simulink model "SysGenBCM1CoreV2"  (R2015b)
settings: Solver=ode45  StartTime=0.0  StopTime=2e-3  MaxStep=100e-6  RelTol=1e-3
undefined symbols (not defined in the file): AXI4, Lite
libraries: xbsIndex_r4 x94
settings Model: DataTypeOverride=Double  MinMaxOverflowLogging=MinMaxAndOverflow  FPTRunName=DoubleOverride  Creator=ssmith  LastModifiedBy=leosap
settings DataIOCC: SaveFormat=Array
settings DebuggingCC: UnderspecifiedInitializationDetection=Classic  MergeDetectMultiDrivingBlocksExec=none  SolverPrmCheckMsg=warning
settings HardwareCC: ProdBitPerPointer=32  ProdLargestAtomicFloat=None  ProdIntDivRoundTo=Undefined  ProdEndianess=Unspecified  ProdWordSize=32  ProdHWDeviceType=32-bit Generic
settings GRTTargetCC: GeneratePreprocessorConditionals=Disable all
settings ConfigComp: CovModelRefEnable=Off  CovSFcnEnable=off

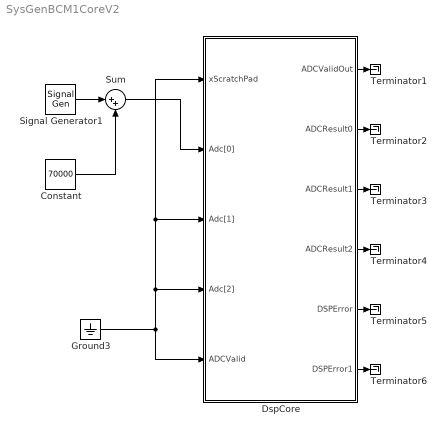
== system SysGenBCM1CoreV2 ==
  Constant : Constant  Value=70000
  DspCore : Subsystem
  Ground3 : Ground
  Signal Generator1 : SignalGenerator  Amplitude=65000  Frequency=1E+6  Units=rad/sec
  Sum : Sum  Inputs=|++
  Terminator{1..6} (6 alike) : Terminator
  wires:
  Ground3/1 -> DspCore/5(ADCValid), DspCore/3(Adc[1]), DspCore/1(xScratchPad), DspCore/4(Adc[2])
  Constant/1 -> Sum/2
  Signal Generator1/1 -> Sum/1
  DspCore/1(ADCValidOut) -> Terminator1/1
  DspCore/2(ADCResult0) -> Terminator2/1
  DspCore/3(ADCResult1) -> Terminator3/1
  DspCore/4(ADCResult2) -> Terminator4/1
  DspCore/5(DSPError) -> Terminator5/1
  DspCore/6(DSPError1) -> Terminator6/1
  Sum/1 -> DspCore/2(Adc[0])

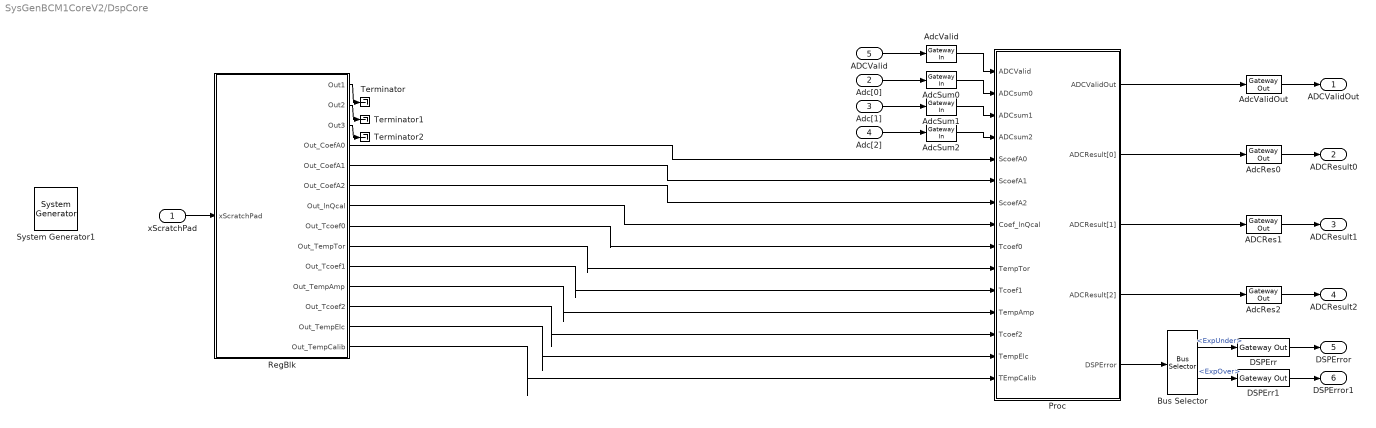
== system SysGenBCM1CoreV2/DspCore ==
  xScratchPad : Inport
  Adc[0] : Inport  Port=2
  Adc[1] : Inport  Port=3
  Adc[2] : Inport  Port=4
  ADCValid : Inport  Port=5
  " System Generator1" : xbsIndex_r4/ System Generator  Tag=genX  xilinxfamily=kintexu  part=xcku040  speed=-2-e  package=ffva1156  synthesis_tool=Vivado  clock_wrapper=Clock Enables  directory=./netlist  proj_type=Vivado  Synth_file=Vivado Synthesis Defaults  Impl_file=Vivado Implementation Defaults  testbench=off  simulink_period=5.385e-9  sysclk_period=5.385  dcm_input_clock_period=10  incr_netlist=off  trim_vbits=Everywhere in SubSystem  dbl_ovrd=According to Block Masks  core_generation=According to Block Masks  run_coregen=off  deprecated_control=off  eval_field=0  block_type=sysgen
  ADCRes1 : xbsIndex_r4/Gateway Out  inherit_from_input=on  hdl_port=on  rows=1  columns=1  UseAsDAC=off  DACChannel='1'  interface=None  automatic_assignment=on  address_offset=hex2dec('00')  intf_name=''  intf_description=''  timing_constraint=None  locs_specified=off  LOCs={}  io_standard={}  block_type=gatewayout
  AdcRes0 : xbsIndex_r4/Gateway Out  inherit_from_input=on  hdl_port=on  rows=1  columns=1  UseAsDAC=off  DACChannel='1'  interface=None  automatic_assignment=on  address_offset=hex2dec('00')  intf_name=''  intf_description=''  timing_constraint=None  locs_specified=off  LOCs={}  io_standard={}  block_type=gatewayout
  AdcRes2 : xbsIndex_r4/Gateway Out  inherit_from_input=on  hdl_port=on  rows=1  columns=1  UseAsDAC=off  DACChannel='1'  interface=None  automatic_assignment=on  address_offset=hex2dec('00')  intf_name=''  intf_description=''  timing_constraint=None  locs_specified=off  LOCs={}  io_standard={}  block_type=gatewayout
  AdcSum0 : xbsIndex_r4/Gateway In  gui_display_data_type=Fixed-point  arith_type=Unsigned  n_bits=32  bin_pt=0  preci_type=Single  exp_width=8  frac_width=24  rows=1  columns=1  quantization="Round  (unbiased: +/- Inf)"  overflow=Saturate  period=5.385E-9  UseAsADC=off  ADCChannel='1'  interface=None  automatic_assignment=on  address_offset=hex2dec('00')  intf_name=''  intf_description=''  default_value=0  timing_constraint=None  locs_specified=off  LOCs={}  io_standard={}  inherit_from_input=off  hdl_port=on  dbl_ovrd=off  block_type=gatewayin
  AdcSum1 : xbsIndex_r4/Gateway In  gui_display_data_type=Fixed-point  arith_type=Unsigned  n_bits=32  bin_pt=0  preci_type=Single  exp_width=8  frac_width=24  rows=1  columns=1  quantization="Round  (unbiased: +/- Inf)"  overflow=Saturate  period=5.385E-9  UseAsADC=off  ADCChannel='1'  interface=None  automatic_assignment=on  address_offset=hex2dec('00')  intf_name=''  intf_description=''  default_value=0  timing_constraint=None  locs_specified=off  LOCs={}  io_standard={}  inherit_from_input=off  hdl_port=on  dbl_ovrd=off  block_type=gatewayin
  AdcSum2 : xbsIndex_r4/Gateway In  gui_display_data_type=Fixed-point  arith_type=Unsigned  n_bits=32  bin_pt=0  preci_type=Single  exp_width=8  frac_width=24  rows=1  columns=1  quantization="Round  (unbiased: +/- Inf)"  overflow=Saturate  period=5.385E-9  UseAsADC=off  ADCChannel='1'  interface=None  automatic_assignment=on  address_offset=hex2dec('00')  intf_name=''  intf_description=''  default_value=0  timing_constraint=None  locs_specified=off  LOCs={}  io_standard={}  inherit_from_input=off  hdl_port=on  dbl_ovrd=off  block_type=gatewayin
  AdcValid : xbsIndex_r4/Gateway In  gui_display_data_type=Boolean  arith_type=Boolean  n_bits=1  bin_pt=0  preci_type=Single  exp_width=8  frac_width=24  rows=1  columns=1  quantization="Round  (unbiased: +/- Inf)"  overflow=Saturate  period=5.385E-9  UseAsADC=off  ADCChannel='1'  interface=None  automatic_assignment=on  address_offset=hex2dec('00')  intf_name=''  intf_description=''  default_value=0  timing_constraint=None  locs_specified=off  LOCs={}  io_standard={}  inherit_from_input=off  hdl_port=on  dbl_ovrd=off  block_type=gatewayin
  AdcValidOut : xbsIndex_r4/Gateway Out  inherit_from_input=on  hdl_port=on  rows=1  columns=1  UseAsDAC=off  DACChannel='1'  interface=None  automatic_assignment=on  address_offset=hex2dec('00')  intf_name=''  intf_description=''  timing_constraint=None  locs_specified=off  LOCs={}  io_standard={}  block_type=gatewayout
  Bus Selector : BusSelector  OutputSignals=ExpUnder,ExpOver
  DSPErr : xbsIndex_r4/Gateway Out  inherit_from_input=on  hdl_port=on  rows=1  columns=1  UseAsDAC=off  DACChannel='1'  interface=None  automatic_assignment=on  address_offset=hex2dec('00')  intf_name=''  intf_description=''  timing_constraint=None  locs_specified=off  LOCs={}  io_standard={}  block_type=gatewayout
  DSPErr1 : xbsIndex_r4/Gateway Out  inherit_from_input=on  hdl_port=on  rows=1  columns=1  UseAsDAC=off  DACChannel='1'  interface=None  automatic_assignment=on  address_offset=hex2dec('00')  intf_name=''  intf_description=''  timing_constraint=None  locs_specified=off  LOCs={}  io_standard={}  block_type=gatewayout
  Proc : Subsystem
  RegBlk : Subsystem
  Terminator : Terminator
  Terminator1 : Terminator
  Terminator2 : Terminator
  ADCValidOut : Outport
  ADCResult0 : Outport  Port=2
  ADCResult1 : Outport  Port=3
  ADCResult2 : Outport  Port=4
  DSPError : Outport  Port=5
  DSPError1 : Outport  Port=6
  wires:
  xScratchPad/1 -> RegBlk/1(xScratchPad)
  Proc/1(ADCValidOut) -> AdcValidOut/1
  Adc[2]/1 -> AdcSum2/1
  Adc[1]/1 -> AdcSum1/1
  Adc[0]/1 -> AdcSum0/1
  Proc/3(ADCResult[1]) -> ADCRes1/1
  Proc/4(ADCResult[2]) -> AdcRes2/1
  Proc/2(ADCResult[0]) -> AdcRes0/1
  ADCValid/1 -> AdcValid/1
  AdcRes0/1 -> ADCResult0/1
  AdcRes2/1 -> ADCResult2/1
  ADCRes1/1 -> ADCResult1/1
  AdcValidOut/1 -> ADCValidOut/1
  AdcValid/1 -> Proc/1(ADCValid)
  AdcSum2/1 -> Proc/4(ADCsum2)
  AdcSum1/1 -> Proc/3(ADCsum1)
  AdcSum0/1 -> Proc/2(ADCsum0)
  DSPErr/1 -> DSPError/1
  Proc/5(DSPError) -> Bus Selector/1
  Bus Selector/1 -> DSPErr/1  "<ExpUnder>"
  DSPErr1/1 -> DSPError1/1
  Bus Selector/2 -> DSPErr1/1  "<ExpOver>"
  RegBlk/4(Out_CoefA0) -> Proc/5(ScoefA0)
  RegBlk/5(Out_CoefA1) -> Proc/6(ScoefA1)
  RegBlk/6(Out_CoefA2) -> Proc/7(ScoefA2)
  RegBlk/7(Out_lnQcal) -> Proc/8(Coef_lnQcal)
  RegBlk/8(Out_Tcoef0) -> Proc/9(Tcoef0)
  RegBlk/13(Out_TempElc) -> Proc/14(TempElc)
  RegBlk/12(Out_Tcoef2) -> Proc/13(Tcoef2)
  RegBlk/11(Out_TempAmp) -> Proc/12(TempAmp)
  RegBlk/10(Out_Tcoef1) -> Proc/11(Tcoef1)
  RegBlk/9(Out_TempTor) -> Proc/10(TempTor)
  RegBlk/14(Out_TempCalib) -> Proc/15(TEmpCalib)
  RegBlk/1(Out1) -> Terminator/1
  RegBlk/2(Out2) -> Terminator1/1
  RegBlk/3(Out3) -> Terminator2/1

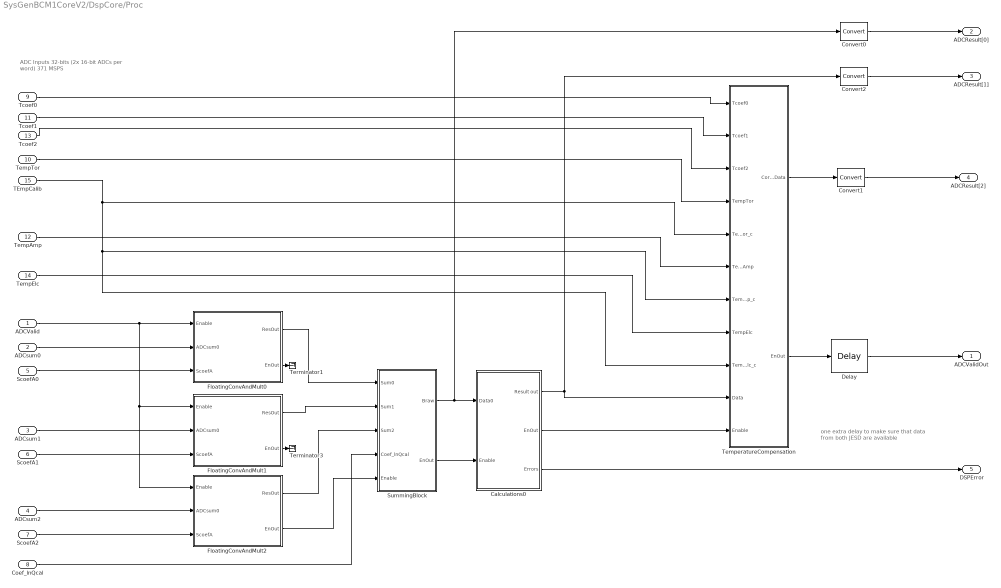
== system SysGenBCM1CoreV2/DspCore/Proc ==
  note: ADC Inputs
      | 32-bits (2x 16-bit ADCs per word)
      | 371 MSPS
  note: one extra delay to make sure that data from both JESD are available
  ADCValid : Inport
  ADCsum0 : Inport  Port=2
  ADCsum1 : Inport  Port=3
  ADCsum2 : Inport  Port=4
  ScoefA0 : Inport  Port=5  SampleTime=5.385E-9
  ScoefA1 : Inport  Port=6  SampleTime=5.385E-9
  ScoefA2 : Inport  Port=7  SampleTime=5.385E-9
  Coef_lnQcal : Inport  Port=8  SampleTime=5.385E-9
  Tcoef0 : Inport  Port=9  SampleTime=5.385E-9
  TempTor : Inport  Port=10  SampleTime=5.385E-9
  Tcoef1 : Inport  Port=11  SampleTime=5.385E-9
  TempAmp : Inport  Port=12  SampleTime=5.385E-9
  Tcoef2 : Inport  Port=13  SampleTime=5.385E-9
  TempElc : Inport  Port=14  SampleTime=5.385E-9
  TEmpCalib : Inport  Port=15  SampleTime=5.385E-9
  Calculations0 : Subsystem
  Convert0 : xbsIndex_r4/Convert  gui_display_data_type=Fixed-point  arith_type="Signed  (2's comp)"  n_bits=32  bin_pt=0  float_type=Single  exp_bits=8  fraction_bits=24  quantization="Round  (unbiased: +/- Inf)"  overflow=Saturate  en=off  latency=1  pipeline=off  dbl_ovrd=off  block_type=convert
  Convert1 : xbsIndex_r4/Convert  gui_display_data_type=Fixed-point  arith_type="Signed  (2's comp)"  n_bits=32  bin_pt=0  float_type=Single  exp_bits=8  fraction_bits=24  quantization="Round  (unbiased: +/- Inf)"  overflow=Saturate  en=off  latency=1  pipeline=off  dbl_ovrd=off  block_type=convert
  Convert2 : xbsIndex_r4/Convert  gui_display_data_type=Fixed-point  arith_type="Signed  (2's comp)"  n_bits=32  bin_pt=0  float_type=Single  exp_bits=8  fraction_bits=24  quantization="Round  (unbiased: +/- Inf)"  overflow=Saturate  en=off  latency=1  pipeline=off  dbl_ovrd=off  block_type=convert
  Delay : xbsIndex_r4/Delay  rst=off  infoeditControl=Selection of Reset will increase slice count due to use of real FFs and instead of SRLs  en=off  latency=2  reg_retiming=off  dbl_ovrd=off  block_type=delay
      settings: infoedit=Hardware notes: A delay line is a chain, each link of which is an SRL16 or SRL32 followed by a flip-flop.
  FloatingConvAndMult0 : Subsystem
  FloatingConvAndMult1 : Subsystem
  FloatingConvAndMult2 : Subsystem
  SummingBlock : Subsystem
  TemperatureCompensation : Subsystem
  Terminator1 : Terminator
  Terminator3 : Terminator
  ADCValidOut : Outport
  ADCResult[0] : Outport  Port=2
  ADCResult[1] : Outport  Port=3
  ADCResult[2] : Outport  Port=4
  DSPError : Outport  Port=5
  wires:
  ScoefA0/1 -> FloatingConvAndMult0/3(ScoefA)
  ScoefA1/1 -> FloatingConvAndMult1/3(ScoefA)
  ScoefA2/1 -> FloatingConvAndMult2/3(ScoefA)
  FloatingConvAndMult0/1(ResOut) -> SummingBlock/1(Sum0)
  FloatingConvAndMult1/1(ResOut) -> SummingBlock/2(Sum1)
  FloatingConvAndMult2/1(ResOut) -> SummingBlock/3(Sum2)
  SummingBlock/1(Braw) -> Convert0/1, Calculations0/1(Data0)
  SummingBlock/2(EnOut) -> Calculations0/2(Enable)
  TemperatureCompensation/1(CorrectedData) -> Convert1/1
  ADCsum0/1 -> FloatingConvAndMult0/2(ADCsum0)
  ADCsum1/1 -> FloatingConvAndMult1/2(ADCsum0)
  ADCsum2/1 -> FloatingConvAndMult2/2(ADCsum0)
  ADCValid/1 -> FloatingConvAndMult2/1(Enable), FloatingConvAndMult1/1(Enable), FloatingConvAndMult0/1(Enable)
  FloatingConvAndMult0/2(EnOut) -> Terminator1/1
  FloatingConvAndMult1/2(EnOut) -> Terminator3/1
  Convert0/1 -> ADCResult[0]/1
  Convert1/1 -> ADCResult[2]/1
  FloatingConvAndMult2/2(EnOut) -> SummingBlock/5(Enable)
  Coef_lnQcal/1 -> SummingBlock/4(Coef_lnQcal)
  Calculations0/3(Errors) -> DSPError/1
  TemperatureCompensation/2(EnOut) -> Delay/1
  Calculations0/2(EnOut) -> TemperatureCompensation/11(Enable)
  Delay/1 -> ADCValidOut/1
  Calculations0/1(Result out) -> Convert2/1, TemperatureCompensation/10(Data)
  Convert2/1 -> ADCResult[1]/1
  Tcoef0/1 -> TemperatureCompensation/1(Tcoef0)
  TempTor/1 -> TemperatureCompensation/4(TempTor)
  TempAmp/1 -> TemperatureCompensation/6(TempAmp)
  TempElc/1 -> TemperatureCompensation/8(TempElc)
  Tcoef1/1 -> TemperatureCompensation/2(Tcoef1)
  Tcoef2/1 -> TemperatureCompensation/3(Tcoef2)
  TEmpCalib/1 -> TemperatureCompensation/7(TempAmp_c), TemperatureCompensation/9(TempElc_c), TemperatureCompensation/5(TempTor_c)

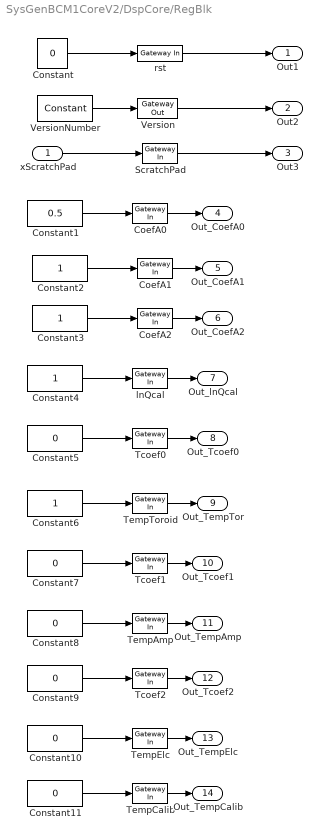
== system SysGenBCM1CoreV2/DspCore/RegBlk ==
  xScratchPad : Inport
  CoefA0 : xbsIndex_r4/Gateway In  gui_display_data_type=Floating-point  arith_type=Floating-point  n_bits=32  bin_pt=31  preci_type=Single  exp_width=8  frac_width=24  rows=1  columns=1  quantization="Round  (unbiased: +/- Inf)"  overflow=Saturate  period=5.385E-9  UseAsADC=off  ADCChannel='1'  interface=AXI4-Lite  automatic_assignment=off  address_offset=hex2dec('004')  intf_name='rwreg'  intf_description=''  default_value=hex2dec('3f800000')  timing_constraint=None  locs_specified=off  LOCs={}  io_standard={}  inherit_from_input=off  hdl_port=on  dbl_ovrd=off  block_type=gatewayin
  CoefA1 : xbsIndex_r4/Gateway In  gui_display_data_type=Floating-point  arith_type=Floating-point  n_bits=32  bin_pt=0  preci_type=Single  exp_width=8  frac_width=24  rows=1  columns=1  quantization="Round  (unbiased: +/- Inf)"  overflow=Saturate  period=5.385E-9  UseAsADC=off  ADCChannel='1'  interface=AXI4-Lite  automatic_assignment=off  address_offset=hex2dec('008')  intf_name='rwreg'  intf_description=''  default_value=hex2dec('3f800001')  timing_constraint=None  locs_specified=off  LOCs={}  io_standard={}  inherit_from_input=off  hdl_port=on  dbl_ovrd=off  block_type=gatewayin
  CoefA2 : xbsIndex_r4/Gateway In  gui_display_data_type=Floating-point  arith_type=Floating-point  n_bits=32  bin_pt=0  preci_type=Single  exp_width=8  frac_width=24  rows=1  columns=1  quantization="Round  (unbiased: +/- Inf)"  overflow=Saturate  period=5.385E-9  UseAsADC=off  ADCChannel='1'  interface=AXI4-Lite  automatic_assignment=off  address_offset=hex2dec('00C')  intf_name='rwreg'  intf_description=''  default_value=hex2dec('3f800002')  timing_constraint=None  locs_specified=off  LOCs={}  io_standard={}  inherit_from_input=off  hdl_port=on  dbl_ovrd=off  block_type=gatewayin
  Constant{,5,7..11} (7 alike) : Constant  Value=0
  Constant1 : Constant  Value=0.5
  Constant{2..4,6} (4 alike) : Constant
  ScratchPad : xbsIndex_r4/Gateway In  gui_display_data_type=Fixed-point  arith_type="Signed  (2's comp)"  n_bits=32  bin_pt=0  preci_type=Single  exp_width=8  frac_width=24  rows=1  columns=1  quantization="Round  (unbiased: +/- Inf)"  overflow=Saturate  period=5.385e-9  UseAsADC=off  ADCChannel='1'  interface=AXI4-Lite  automatic_assignment=off  address_offset=hex2dec('FFC')  intf_name=''  intf_description=''  default_value=0  timing_constraint=None  locs_specified=off  LOCs={}  io_standard={}  inherit_from_input=off  hdl_port=on  dbl_ovrd=off  block_type=gatewayin
  Tcoef0 : xbsIndex_r4/Gateway In  gui_display_data_type=Floating-point  arith_type=Floating-point  n_bits=32  bin_pt=0  preci_type=Single  exp_width=8  frac_width=24  rows=1  columns=1  quantization="Round  (unbiased: +/- Inf)"  overflow=Saturate  period=5.385E-9  UseAsADC=off  ADCChannel='1'  interface=AXI4-Lite  automatic_assignment=off  address_offset=hex2dec('014')  intf_name='rwreg'  intf_description=''  default_value=0  timing_constraint=None  locs_specified=off  LOCs={}  io_standard={}  inherit_from_input=off  hdl_port=on  dbl_ovrd=off  block_type=gatewayin
  Tcoef1 : xbsIndex_r4/Gateway In  gui_display_data_type=Floating-point  arith_type=Floating-point  n_bits=32  bin_pt=0  preci_type=Single  exp_width=8  frac_width=24  rows=1  columns=1  quantization="Round  (unbiased: +/- Inf)"  overflow=Saturate  period=5.385E-9  UseAsADC=off  ADCChannel='1'  interface=AXI4-Lite  automatic_assignment=off  address_offset=hex2dec('01C')  intf_name='rwreg'  intf_description=''  default_value=0  timing_constraint=None  locs_specified=off  LOCs={}  io_standard={}  inherit_from_input=off  hdl_port=on  dbl_ovrd=off  block_type=gatewayin
  Tcoef2 : xbsIndex_r4/Gateway In  gui_display_data_type=Floating-point  arith_type=Floating-point  n_bits=32  bin_pt=0  preci_type=Single  exp_width=8  frac_width=24  rows=1  columns=1  quantization="Round  (unbiased: +/- Inf)"  overflow=Saturate  period=5.385E-9  UseAsADC=off  ADCChannel='1'  interface=AXI4-Lite  automatic_assignment=off  address_offset=hex2dec('024')  intf_name='rwreg'  intf_description=''  default_value=0  timing_constraint=None  locs_specified=off  LOCs={}  io_standard={}  inherit_from_input=off  hdl_port=on  dbl_ovrd=off  block_type=gatewayin
  TempAmp : xbsIndex_r4/Gateway In  gui_display_data_type=Floating-point  arith_type=Floating-point  n_bits=32  bin_pt=0  preci_type=Single  exp_width=8  frac_width=24  rows=1  columns=1  quantization="Round  (unbiased: +/- Inf)"  overflow=Saturate  period=5.385E-9  UseAsADC=off  ADCChannel='1'  interface=AXI4-Lite  automatic_assignment=off  address_offset=hex2dec('020')  intf_name='rwreg'  intf_description=''  default_value=0  timing_constraint=None  locs_specified=off  LOCs={}  io_standard={}  inherit_from_input=off  hdl_port=on  dbl_ovrd=off  block_type=gatewayin
  TempCalib : xbsIndex_r4/Gateway In  gui_display_data_type=Floating-point  arith_type=Floating-point  n_bits=32  bin_pt=0  preci_type=Single  exp_width=8  frac_width=24  rows=1  columns=1  quantization="Round  (unbiased: +/- Inf)"  overflow=Saturate  period=5.385E-9  UseAsADC=off  ADCChannel='1'  interface=AXI4-Lite  automatic_assignment=off  address_offset=hex2dec('02c')  intf_name='rwreg'  intf_description=''  default_value=hex2dec('43941333')  timing_constraint=None  locs_specified=off  LOCs={}  io_standard={}  inherit_from_input=off  hdl_port=on  dbl_ovrd=off  block_type=gatewayin
  TempElc : xbsIndex_r4/Gateway In  gui_display_data_type=Floating-point  arith_type=Floating-point  n_bits=32  bin_pt=0  preci_type=Single  exp_width=8  frac_width=24  rows=1  columns=1  quantization="Round  (unbiased: +/- Inf)"  overflow=Saturate  period=5.385E-9  UseAsADC=off  ADCChannel='1'  interface=AXI4-Lite  automatic_assignment=off  address_offset=hex2dec('028')  intf_name='rwreg'  intf_description=''  default_value=0  timing_constraint=None  locs_specified=off  LOCs={}  io_standard={}  inherit_from_input=off  hdl_port=on  dbl_ovrd=off  block_type=gatewayin
  TempToroid : xbsIndex_r4/Gateway In  gui_display_data_type=Floating-point  arith_type=Floating-point  n_bits=32  bin_pt=0  preci_type=Single  exp_width=8  frac_width=24  rows=1  columns=1  quantization="Round  (unbiased: +/- Inf)"  overflow=Saturate  period=5.385E-9  UseAsADC=off  ADCChannel='1'  interface=AXI4-Lite  automatic_assignment=off  address_offset=hex2dec('018')  intf_name='rwreg'  intf_description=''  default_value=0  timing_constraint=None  locs_specified=off  LOCs={}  io_standard={}  inherit_from_input=off  hdl_port=on  dbl_ovrd=off  block_type=gatewayin
  Version : xbsIndex_r4/Gateway Out  inherit_from_input=on  hdl_port=on  rows=1  columns=1  UseAsDAC=off  DACChannel='1'  interface=AXI4-Lite  automatic_assignment=off  address_offset=hex2dec('000')  intf_name='rwreg'  intf_description=''  timing_constraint=None  locs_specified=off  LOCs={}  io_standard={}  block_type=gatewayout
  VersionNumber : xbsIndex_r4/Constant  const=hex2dec('00000001')  gui_display_data_type=Fixed-point  arith_type=Unsigned  n_bits=32  bin_pt=0  preci_type=Single  exp_width=8  frac_width=24  explicit_period=off  period=1  equ=P=C  opselect=C  inp2=PCIN>>17  opr=+  inp1=P  carry=CIN  dbl_ovrd=off  block_type=constant
  lnQcal : xbsIndex_r4/Gateway In  gui_display_data_type=Floating-point  arith_type=Floating-point  n_bits=32  bin_pt=0  preci_type=Single  exp_width=8  frac_width=24  rows=1  columns=1  quantization="Round  (unbiased: +/- Inf)"  overflow=Saturate  period=5.385E-9  UseAsADC=off  ADCChannel='1'  interface=AXI4-Lite  automatic_assignment=off  address_offset=hex2dec('010')  intf_name='rwreg'  intf_description=''  default_value=0  timing_constraint=None  locs_specified=off  LOCs={}  io_standard={}  inherit_from_input=off  hdl_port=on  dbl_ovrd=off  block_type=gatewayin
  rst : xbsIndex_r4/Gateway In  gui_display_data_type=Boolean  arith_type=Boolean  n_bits=16  bin_pt=14  preci_type=Single  exp_width=8  frac_width=24  rows=1  columns=1  quantization="Round  (unbiased: +/- Inf)"  overflow=Saturate  period=5.385e-9  UseAsADC=off  ADCChannel='1'  interface=None  automatic_assignment=on  address_offset=hex2dec('00')  intf_name=''  intf_description=''  default_value=0  timing_constraint=None  locs_specified=off  LOCs={}  io_standard={}  inherit_from_input=off  hdl_port=on  dbl_ovrd=off  block_type=gatewayin
  Out1 : Outport
  Out2 : Outport  Port=2
  Out3 : Outport  Port=3
  Out_CoefA0 : Outport  Port=4
  Out_CoefA1 : Outport  Port=5
  Out_CoefA2 : Outport  Port=6
  Out_lnQcal : Outport  Port=7
  Out_Tcoef0 : Outport  Port=8
  Out_TempTor : Outport  Port=9
  Out_Tcoef1 : Outport  Port=10
  Out_TempAmp : Outport  Port=11
  Out_Tcoef2 : Outport  Port=12
  Out_TempElc : Outport  Port=13
  Out_TempCalib : Outport  Port=14
  wires:
  Constant/1 -> rst/1
  ScratchPad/1 -> Out3/1
  Version/1 -> Out2/1
  rst/1 -> Out1/1
  xScratchPad/1 -> ScratchPad/1
  VersionNumber/1 -> Version/1
  Constant1/1 -> CoefA0/1
  CoefA0/1 -> Out_CoefA0/1
  Constant2/1 -> CoefA1/1
  CoefA1/1 -> Out_CoefA1/1
  Constant3/1 -> CoefA2/1
  CoefA2/1 -> Out_CoefA2/1
  Constant4/1 -> lnQcal/1
  lnQcal/1 -> Out_lnQcal/1
  Constant5/1 -> Tcoef0/1
  Constant6/1 -> TempToroid/1
  Constant7/1 -> Tcoef1/1
  Constant8/1 -> TempAmp/1
  Constant9/1 -> Tcoef2/1
  Constant10/1 -> TempElc/1
  TempToroid/1 -> Out_TempTor/1
  Tcoef0/1 -> Out_Tcoef0/1
  Tcoef2/1 -> Out_Tcoef2/1
  TempElc/1 -> Out_TempElc/1
  Tcoef1/1 -> Out_Tcoef1/1
  TempAmp/1 -> Out_TempAmp/1
  Constant11/1 -> TempCalib/1
  TempCalib/1 -> Out_TempCalib/1

== system SysGenBCM1CoreV2/DspCore/Proc/Calculations0 ==
  note: Q_in = Q_cal*(Real losses/calib Loses)*10^(Braw/Ucal)
      | Rewrite
      | Q_in = exp^(lnQcal*(Real loses/calib loses)  + Braw*(ln10/Ucal))
      | Or
      | Q_in= exp^Braw_new
      |
      | BRaw=SUM0(ADC(i))*A0+ SUM1(ADC(i))*A1 +SUM2(ADC(i))*A2
      | SUms done outside of core
      |
      | Braw_new = SUM0(ADC(i))*A0_new+ SUM1(ADC(i))*A1_new +SUM2(ADC(i))*A2_new + CoefB
      |
      | A0_new = A0 *(ln10/Ucal)
      | A1_new = A1 *(ln10/Ucal)
      | A2_new = A2 *(ln10/Ucal)
      | CoefB = ln(Qcal*(Real_loses/Calib/loses))
      | All coef are float 32
  Data0 : Inport
  Enable : Inport  Port=2
  Add : xbsIndex_r4/Gateway Out  inherit_from_input=on  hdl_port=on  rows=1  columns=1  UseAsDAC=off  DACChannel='1'  interface=AXI4-Lite  automatic_assignment=off  address_offset=hex2dec('118')  intf_name=''  intf_description=''  timing_constraint=None  locs_specified=off  LOCs={}  io_standard={}  block_type=gatewayout
  Bus Creator : BusCreator  Inputs=2
  Delay1 : xbsIndex_r4/Delay  rst=off  infoeditControl=Selection of Reset will increase slice count due to use of real FFs and instead of SRLs  en=off  latency=7  reg_retiming=off  dbl_ovrd=off  block_type=delay
      settings: infoedit=Hardware notes: A delay line is a chain, each link of which is an SRL16 or SRL32 followed by a flip-flop.
  Exponential1 : xbsIndex_r4/Exponential  flow_control=NonBlocking  axi_optimize_goal=Resources  bmg_use=FullUsage  latency=7  has_a_tlast=off  has_a_tuser=off  en=on  has_result_tready=off  has_underflow=on  has_overflow=on  fpo_op_type=exponential  rate=1  has_b_tlast=false  has_b_tuser=false  result_tlast_behv=1  has_divide_by_zero=false  has_invalid_op=false  block_type=exponential
      settings: infoedit=Blocking: Wait for data on all inputs, allow back-pressure.<br>NonBlocking: operate every cycle in which all inputs are valid, no back-pressure.
  Terminator6 : Terminator
  Result out : Outport
  EnOut : Outport  Port=2
  Errors : Outport  Port=3
  wires:
  Data0/1 -> Exponential1/1
  Enable/1 -> Delay1/1, Exponential1/2
  Exponential1/1 -> Result out/1, Add/1
  Exponential1/3 -> Bus Creator/2  "ExpOver"
  Bus Creator/1 -> Errors/1
  Exponential1/2 -> Bus Creator/1  "ExpUnder"
  Add/1 -> Terminator6/1
  Delay1/1 -> EnOut/1

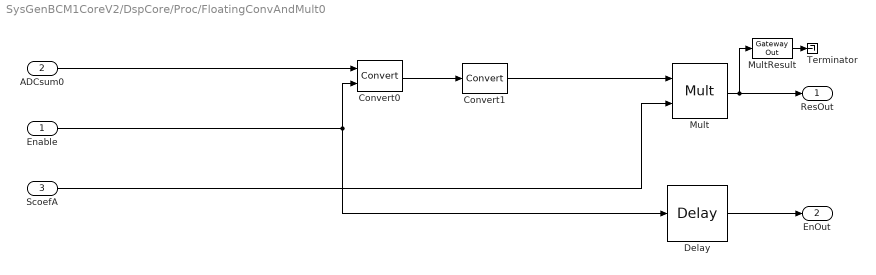
== system SysGenBCM1CoreV2/DspCore/Proc/FloatingConvAndMult0 ==
  Enable : Inport  SampleTime=5.385E-9
  ADCsum0 : Inport  Port=2
  ScoefA : Inport  Port=3  SampleTime=5.385E-9
  Convert0 : xbsIndex_r4/Convert  gui_display_data_type=Fixed-point  arith_type="Signed  (2's comp)"  n_bits=32  bin_pt=0  float_type=Single  exp_bits=8  fraction_bits=24  quantization=Truncate  overflow=Wrap  en=on  latency=1  pipeline=off  dbl_ovrd=off  block_type=convert
  Convert1 : xbsIndex_r4/Convert  gui_display_data_type=Floating-point  arith_type=Floating-point  n_bits=16  bin_pt=14  float_type=Single  exp_bits=8  fraction_bits=24  quantization=Truncate  overflow=Wrap  en=off  latency=1  pipeline=off  dbl_ovrd=off  block_type=convert
  Delay : xbsIndex_r4/Delay  rst=off  infoeditControl=Selection of Reset will increase slice count due to use of real FFs and instead of SRLs  en=off  latency=6  reg_retiming=off  dbl_ovrd=off  block_type=delay
      settings: infoedit=Hardware notes: A delay line is a chain, each link of which is an SRL16 or SRL32 followed by a flip-flop.
  Mult : xbsIndex_r4/Mult  precision=Full  arith_type="Signed  (2's comp)"  n_bits=16  bin_pt=14  quantization=Truncate  overflow=Wrap  en=off  latency=4  use_behavioral_HDL=off  opt=Speed  use_embedded=on  optimum_pipeline=off  pipeline=on  dbl_ovrd=off  use_rpm=on  placement_style=Triangular  block_type=mult
  MultResult : xbsIndex_r4/Gateway Out  inherit_from_input=on  hdl_port=on  rows=1  columns=1  UseAsDAC=off  DACChannel='1'  interface=AXI4-Lite  automatic_assignment=off  address_offset=hex2dec('100')  intf_name=''  intf_description=''  timing_constraint=None  locs_specified=off  LOCs={}  io_standard={}  block_type=gatewayout
  Terminator : Terminator
  ResOut : Outport
  EnOut : Outport  Port=2
  wires:
  Mult/1 -> MultResult/1, ResOut/1
  Convert0/1 -> Convert1/1
  Enable/1 -> Delay/1, Convert0/2
  ScoefA/1 -> Mult/2
  Convert1/1 -> Mult/1
  Delay/1 -> EnOut/1
  ADCsum0/1 -> Convert0/1
  MultResult/1 -> Terminator/1

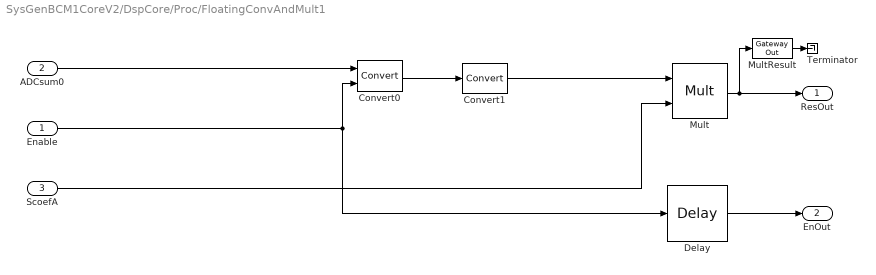
== system SysGenBCM1CoreV2/DspCore/Proc/FloatingConvAndMult1 ==
  Enable : Inport  SampleTime=5.385E-9
  ADCsum0 : Inport  Port=2
  ScoefA : Inport  Port=3  SampleTime=5.385E-9
  Convert0 : xbsIndex_r4/Convert  gui_display_data_type=Fixed-point  arith_type="Signed  (2's comp)"  n_bits=32  bin_pt=0  float_type=Single  exp_bits=8  fraction_bits=24  quantization=Truncate  overflow=Wrap  en=on  latency=1  pipeline=off  dbl_ovrd=off  block_type=convert
  Convert1 : xbsIndex_r4/Convert  gui_display_data_type=Floating-point  arith_type=Floating-point  n_bits=16  bin_pt=14  float_type=Single  exp_bits=8  fraction_bits=24  quantization=Truncate  overflow=Wrap  en=off  latency=1  pipeline=off  dbl_ovrd=off  block_type=convert
  Delay : xbsIndex_r4/Delay  rst=off  infoeditControl=Selection of Reset will increase slice count due to use of real FFs and instead of SRLs  en=off  latency=6  reg_retiming=off  dbl_ovrd=off  block_type=delay
      settings: infoedit=Hardware notes: A delay line is a chain, each link of which is an SRL16 or SRL32 followed by a flip-flop.
  Mult : xbsIndex_r4/Mult  precision=Full  arith_type="Signed  (2's comp)"  n_bits=16  bin_pt=14  quantization=Truncate  overflow=Wrap  en=off  latency=4  use_behavioral_HDL=off  opt=Speed  use_embedded=on  optimum_pipeline=off  pipeline=on  dbl_ovrd=off  use_rpm=on  placement_style=Triangular  block_type=mult
  MultResult : xbsIndex_r4/Gateway Out  inherit_from_input=on  hdl_port=on  rows=1  columns=1  UseAsDAC=off  DACChannel='1'  interface=AXI4-Lite  automatic_assignment=off  address_offset=hex2dec('104')  intf_name=''  intf_description=''  timing_constraint=None  locs_specified=off  LOCs={}  io_standard={}  block_type=gatewayout
  Terminator : Terminator
  ResOut : Outport
  EnOut : Outport  Port=2
  wires:
  Mult/1 -> MultResult/1, ResOut/1
  Convert0/1 -> Convert1/1
  Enable/1 -> Delay/1, Convert0/2
  ScoefA/1 -> Mult/2
  Convert1/1 -> Mult/1
  Delay/1 -> EnOut/1
  ADCsum0/1 -> Convert0/1
  MultResult/1 -> Terminator/1

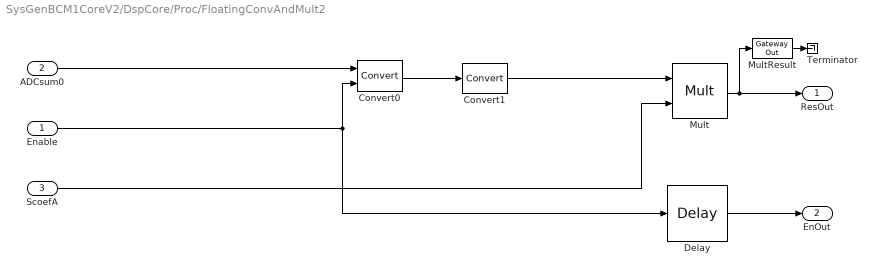
== system SysGenBCM1CoreV2/DspCore/Proc/FloatingConvAndMult2 ==
  Enable : Inport  SampleTime=5.385E-9
  ADCsum0 : Inport  Port=2
  ScoefA : Inport  Port=3  SampleTime=5.385E-9
  Convert0 : xbsIndex_r4/Convert  gui_display_data_type=Fixed-point  arith_type="Signed  (2's comp)"  n_bits=32  bin_pt=0  float_type=Single  exp_bits=8  fraction_bits=24  quantization=Truncate  overflow=Wrap  en=on  latency=1  pipeline=off  dbl_ovrd=off  block_type=convert
  Convert1 : xbsIndex_r4/Convert  gui_display_data_type=Floating-point  arith_type=Floating-point  n_bits=16  bin_pt=14  float_type=Single  exp_bits=8  fraction_bits=24  quantization=Truncate  overflow=Wrap  en=off  latency=1  pipeline=off  dbl_ovrd=off  block_type=convert
  Delay : xbsIndex_r4/Delay  rst=off  infoeditControl=Selection of Reset will increase slice count due to use of real FFs and instead of SRLs  en=off  latency=6  reg_retiming=off  dbl_ovrd=off  block_type=delay
      settings: infoedit=Hardware notes: A delay line is a chain, each link of which is an SRL16 or SRL32 followed by a flip-flop.
  Mult : xbsIndex_r4/Mult  precision=Full  arith_type="Signed  (2's comp)"  n_bits=16  bin_pt=14  quantization=Truncate  overflow=Wrap  en=off  latency=4  use_behavioral_HDL=off  opt=Speed  use_embedded=on  optimum_pipeline=off  pipeline=on  dbl_ovrd=off  use_rpm=on  placement_style=Triangular  block_type=mult
  MultResult : xbsIndex_r4/Gateway Out  inherit_from_input=on  hdl_port=on  rows=1  columns=1  UseAsDAC=off  DACChannel='1'  interface=AXI4-Lite  automatic_assignment=off  address_offset=hex2dec('108')  intf_name=''  intf_description=''  timing_constraint=None  locs_specified=off  LOCs={}  io_standard={}  block_type=gatewayout
  Terminator : Terminator
  ResOut : Outport
  EnOut : Outport  Port=2
  wires:
  Mult/1 -> MultResult/1, ResOut/1
  Convert0/1 -> Convert1/1
  Enable/1 -> Delay/1, Convert0/2
  ScoefA/1 -> Mult/2
  Convert1/1 -> Mult/1
  Delay/1 -> EnOut/1
  ADCsum0/1 -> Convert0/1
  MultResult/1 -> Terminator/1

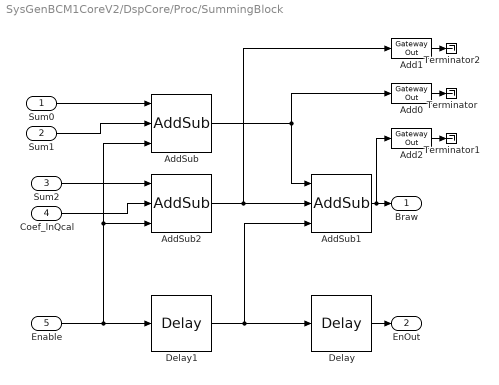
== system SysGenBCM1CoreV2/DspCore/Proc/SummingBlock ==
  Sum0 : Inport
  Sum1 : Inport  Port=2
  Sum2 : Inport  Port=3
  Coef_lnQcal : Inport  Port=4
  Enable : Inport  Port=5
  Add0 : xbsIndex_r4/Gateway Out  inherit_from_input=on  hdl_port=on  rows=1  columns=1  UseAsDAC=off  DACChannel='1'  interface=AXI4-Lite  automatic_assignment=off  address_offset=hex2dec('10C')  intf_name=''  intf_description=''  timing_constraint=None  locs_specified=off  LOCs={}  io_standard={}  block_type=gatewayout
  Add1 : xbsIndex_r4/Gateway Out  inherit_from_input=on  hdl_port=on  rows=1  columns=1  UseAsDAC=off  DACChannel='1'  interface=AXI4-Lite  automatic_assignment=off  address_offset=hex2dec('110')  intf_name=''  intf_description=''  timing_constraint=None  locs_specified=off  LOCs={}  io_standard={}  block_type=gatewayout
  Add2 : xbsIndex_r4/Gateway Out  inherit_from_input=on  hdl_port=on  rows=1  columns=1  UseAsDAC=off  DACChannel='1'  interface=AXI4-Lite  automatic_assignment=off  address_offset=hex2dec('114')  intf_name=''  intf_description=''  timing_constraint=None  locs_specified=off  LOCs={}  io_standard={}  block_type=gatewayout
  AddSub : xbsIndex_r4/AddSub  mode=Addition  use_carryin=off  use_carryout=off  en=on  latency=3  precision=Full  arith_type=Unsigned  n_bits=16  bin_pt=14  quantization=Truncate  overflow=Wrap  use_behavioral_HDL=off  hw_selection=Fabric  pipelined=off  dbl_ovrd=off  block_type=addsub
  AddSub1 : xbsIndex_r4/AddSub  mode=Addition  use_carryin=off  use_carryout=off  en=on  latency=3  precision=Full  arith_type=Unsigned  n_bits=16  bin_pt=14  quantization=Truncate  overflow=Wrap  use_behavioral_HDL=off  hw_selection=Fabric  pipelined=off  dbl_ovrd=off  block_type=addsub
  AddSub2 : xbsIndex_r4/AddSub  mode=Addition  use_carryin=off  use_carryout=off  en=on  latency=3  precision=Full  arith_type=Unsigned  n_bits=16  bin_pt=14  quantization=Truncate  overflow=Wrap  use_behavioral_HDL=off  hw_selection=Fabric  pipelined=off  dbl_ovrd=off  block_type=addsub
  Delay : xbsIndex_r4/Delay  rst=off  infoeditControl=Selection of Reset will increase slice count due to use of real FFs and instead of SRLs  en=off  latency=3  reg_retiming=off  dbl_ovrd=off  block_type=delay
      settings: infoedit=Hardware notes: A delay line is a chain, each link of which is an SRL16 or SRL32 followed by a flip-flop.
  Delay1 : xbsIndex_r4/Delay  rst=off  infoeditControl=Selection of Reset will increase slice count due to use of real FFs and instead of SRLs  en=off  latency=3  reg_retiming=off  dbl_ovrd=off  block_type=delay
      settings: infoedit=Hardware notes: A delay line is a chain, each link of which is an SRL16 or SRL32 followed by a flip-flop.
  Terminator : Terminator
  Terminator1 : Terminator
  Terminator2 : Terminator
  Braw : Outport
  EnOut : Outport  Port=2
  wires:
  AddSub/1 -> AddSub1/1, Add0/1
  AddSub1/1 -> Add2/1, Braw/1
  Delay/1 -> EnOut/1
  Enable/1 -> AddSub2/3, AddSub/3, Delay1/1
  Sum1/1 -> AddSub/2
  Sum0/1 -> AddSub/1
  Delay1/1 -> Delay/1, AddSub1/3
  Add0/1 -> Terminator/1
  Add2/1 -> Terminator1/1
  AddSub2/1 -> Add1/1, AddSub1/2
  Sum2/1 -> AddSub2/1
  Coef_lnQcal/1 -> AddSub2/2
  Add1/1 -> Terminator2/1

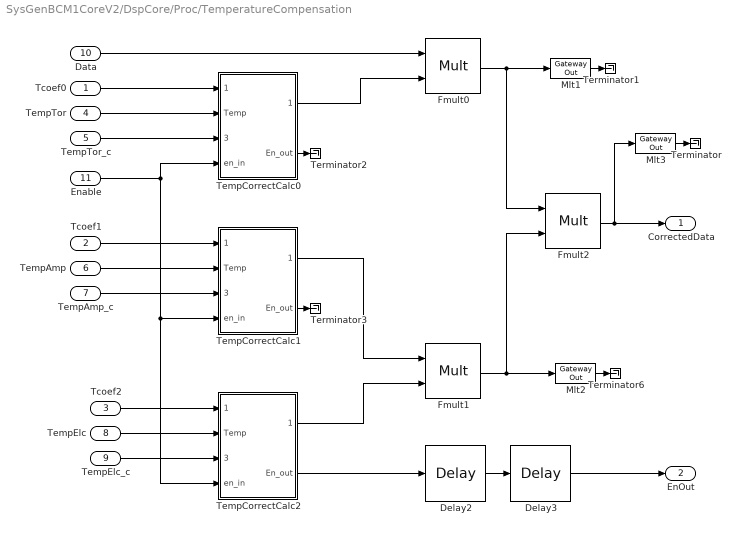
== system SysGenBCM1CoreV2/DspCore/Proc/TemperatureCompensation ==
  Tcoef0 : Inport
  Tcoef1 : Inport  Port=2
  Tcoef2 : Inport  Port=3
  TempTor : Inport  Port=4
  TempTor_c : Inport  Port=5
  TempAmp : Inport  Port=6
  TempAmp_c : Inport  Port=7
  TempElc : Inport  Port=8
  TempElc_c : Inport  Port=9
  Data : Inport  Port=10
  Enable : Inport  Port=11
  Delay2 : xbsIndex_r4/Delay  rst=off  infoeditControl=Selection of Reset will increase slice count due to use of real FFs and instead of SRLs  en=off  latency=4  reg_retiming=off  dbl_ovrd=off  block_type=delay
      settings: infoedit=Hardware notes: A delay line is a chain, each link of which is an SRL16 or SRL32 followed by a flip-flop.
  Delay3 : xbsIndex_r4/Delay  rst=off  infoeditControl=Selection of Reset will increase slice count due to use of real FFs and instead of SRLs  en=off  latency=4  reg_retiming=off  dbl_ovrd=off  block_type=delay
      settings: infoedit=Hardware notes: A delay line is a chain, each link of which is an SRL16 or SRL32 followed by a flip-flop.
  Fmult0 : xbsIndex_r4/Mult  precision=Full  arith_type="Signed  (2's comp)"  n_bits=16  bin_pt=14  quantization=Truncate  overflow=Wrap  en=off  latency=4  use_behavioral_HDL=off  opt=Speed  use_embedded=on  optimum_pipeline=off  pipeline=on  dbl_ovrd=off  use_rpm=on  placement_style=Triangular  block_type=mult
  Fmult1 : xbsIndex_r4/Mult  precision=Full  arith_type="Signed  (2's comp)"  n_bits=16  bin_pt=14  quantization=Truncate  overflow=Wrap  en=off  latency=4  use_behavioral_HDL=off  opt=Speed  use_embedded=on  optimum_pipeline=off  pipeline=on  dbl_ovrd=off  use_rpm=on  placement_style=Triangular  block_type=mult
  Fmult2 : xbsIndex_r4/Mult  precision=Full  arith_type="Signed  (2's comp)"  n_bits=16  bin_pt=14  quantization=Truncate  overflow=Wrap  en=off  latency=4  use_behavioral_HDL=off  opt=Speed  use_embedded=on  optimum_pipeline=off  pipeline=on  dbl_ovrd=off  use_rpm=on  placement_style=Triangular  block_type=mult
  Mlt1 : xbsIndex_r4/Gateway Out  inherit_from_input=on  hdl_port=on  rows=1  columns=1  UseAsDAC=off  DACChannel='1'  interface=AXI4-Lite  automatic_assignment=off  address_offset=hex2dec('140')  intf_name=''  intf_description=''  timing_constraint=None  locs_specified=off  LOCs={}  io_standard={}  block_type=gatewayout
  Mlt2 : xbsIndex_r4/Gateway Out  inherit_from_input=on  hdl_port=on  rows=1  columns=1  UseAsDAC=off  DACChannel='1'  interface=AXI4-Lite  automatic_assignment=off  address_offset=hex2dec('144')  intf_name=''  intf_description=''  timing_constraint=None  locs_specified=off  LOCs={}  io_standard={}  block_type=gatewayout
  Mlt3 : xbsIndex_r4/Gateway Out  inherit_from_input=on  hdl_port=on  rows=1  columns=1  UseAsDAC=off  DACChannel='1'  interface=AXI4-Lite  automatic_assignment=off  address_offset=hex2dec('148')  intf_name=''  intf_description=''  timing_constraint=None  locs_specified=off  LOCs={}  io_standard={}  block_type=gatewayout
  TempCorrectCalc0 : Subsystem
  TempCorrectCalc1 : Subsystem
  TempCorrectCalc2 : Subsystem
  Terminator{,1..3,6} (5 alike) : Terminator
  CorrectedData : Outport
  EnOut : Outport  Port=2
  wires:
  Fmult1/1 -> Fmult2/2, Mlt2/1
  Fmult2/1 -> CorrectedData/1, Mlt3/1
  Delay2/1 -> Delay3/1
  Delay3/1 -> EnOut/1
  Mlt2/1 -> Terminator6/1
  Tcoef0/1 -> TempCorrectCalc0/1(CoefTemp)
  TempTor/1 -> TempCorrectCalc0/2(Temp)
  TempTor_c/1 -> TempCorrectCalc0/3(Temp_c)
  Enable/1 -> TempCorrectCalc0/4(en_in), TempCorrectCalc2/4(en_in), TempCorrectCalc1/4(en_in)
  Tcoef1/1 -> TempCorrectCalc1/1(CoefTemp)
  TempAmp/1 -> TempCorrectCalc1/2(Temp)
  TempAmp_c/1 -> TempCorrectCalc1/3(Temp_c)
  Tcoef2/1 -> TempCorrectCalc2/1(CoefTemp)
  TempElc/1 -> TempCorrectCalc2/2(Temp)
  TempElc_c/1 -> TempCorrectCalc2/3(Temp_c)
  TempCorrectCalc2/1(CorrectOut) -> Fmult1/2
  TempCorrectCalc1/1(CorrectOut) -> Fmult1/1
  Fmult0/1 -> Fmult2/1, Mlt1/1
  Mlt1/1 -> Terminator1/1
  Data/1 -> Fmult0/1
  TempCorrectCalc0/1(CorrectOut) -> Fmult0/2
  TempCorrectCalc2/2(En_out) -> Delay2/1
  Mlt3/1 -> Terminator/1
  TempCorrectCalc0/2(En_out) -> Terminator2/1
  TempCorrectCalc1/2(En_out) -> Terminator3/1

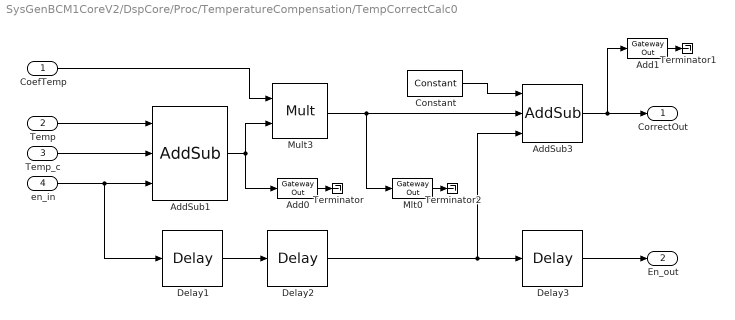
== system SysGenBCM1CoreV2/DspCore/Proc/TemperatureCompensation/TempCorrectCalc0 ==
  CoefTemp : Inport
  Temp : Inport  Port=2
  Temp_c : Inport  Port=3
  en_in : Inport  Port=4
  Add0 : xbsIndex_r4/Gateway Out  inherit_from_input=on  hdl_port=on  rows=1  columns=1  UseAsDAC=off  DACChannel='1'  interface=AXI4-Lite  automatic_assignment=off  address_offset=hex2dec('11C')  intf_name=''  intf_description=''  timing_constraint=None  locs_specified=off  LOCs={}  io_standard={}  block_type=gatewayout
  Add1 : xbsIndex_r4/Gateway Out  inherit_from_input=on  hdl_port=on  rows=1  columns=1  UseAsDAC=off  DACChannel='1'  interface=AXI4-Lite  automatic_assignment=off  address_offset=hex2dec('124')  intf_name=''  intf_description=''  timing_constraint=None  locs_specified=off  LOCs={}  io_standard={}  block_type=gatewayout
  AddSub1 : xbsIndex_r4/AddSub  mode=Subtraction  use_carryin=off  use_carryout=off  en=on  latency=3  precision=Full  arith_type=Unsigned  n_bits=16  bin_pt=14  quantization=Truncate  overflow=Wrap  use_behavioral_HDL=off  hw_selection=Fabric  pipelined=off  dbl_ovrd=off  block_type=addsub
  AddSub3 : xbsIndex_r4/AddSub  mode=Addition  use_carryin=off  use_carryout=off  en=on  latency=2  precision=Full  arith_type=Unsigned  n_bits=16  bin_pt=14  quantization=Truncate  overflow=Wrap  use_behavioral_HDL=off  hw_selection=Fabric  pipelined=off  dbl_ovrd=off  block_type=addsub
  Constant : xbsIndex_r4/Constant  const=1.0  gui_display_data_type=Floating-point  arith_type=Floating-point  n_bits=16  bin_pt=14  preci_type=Single  exp_width=8  frac_width=24  explicit_period=off  period=1  equ=P=C  opselect=C  inp2=PCIN>>17  opr=+  inp1=P  carry=CIN  dbl_ovrd=off  block_type=constant
  Delay1 : xbsIndex_r4/Delay  rst=off  infoeditControl=Selection of Reset will increase slice count due to use of real FFs and instead of SRLs  en=off  latency=3  reg_retiming=off  dbl_ovrd=off  block_type=delay
      settings: infoedit=Hardware notes: A delay line is a chain, each link of which is an SRL16 or SRL32 followed by a flip-flop.
  Delay2 : xbsIndex_r4/Delay  rst=off  infoeditControl=Selection of Reset will increase slice count due to use of real FFs and instead of SRLs  en=off  latency=4  reg_retiming=off  dbl_ovrd=off  block_type=delay
      settings: infoedit=Hardware notes: A delay line is a chain, each link of which is an SRL16 or SRL32 followed by a flip-flop.
  Delay3 : xbsIndex_r4/Delay  rst=off  infoeditControl=Selection of Reset will increase slice count due to use of real FFs and instead of SRLs  en=off  latency=2  reg_retiming=off  dbl_ovrd=off  block_type=delay
      settings: infoedit=Hardware notes: A delay line is a chain, each link of which is an SRL16 or SRL32 followed by a flip-flop.
  Mlt0 : xbsIndex_r4/Gateway Out  inherit_from_input=on  hdl_port=on  rows=1  columns=1  UseAsDAC=off  DACChannel='1'  interface=AXI4-Lite  automatic_assignment=off  address_offset=hex2dec('120')  intf_name=''  intf_description=''  timing_constraint=None  locs_specified=off  LOCs={}  io_standard={}  block_type=gatewayout
  Mult3 : xbsIndex_r4/Mult  precision=Full  arith_type="Signed  (2's comp)"  n_bits=16  bin_pt=14  quantization=Truncate  overflow=Wrap  en=off  latency=4  use_behavioral_HDL=off  opt=Speed  use_embedded=on  optimum_pipeline=off  pipeline=on  dbl_ovrd=off  use_rpm=on  placement_style=Triangular  block_type=mult
  Terminator : Terminator
  Terminator1 : Terminator
  Terminator2 : Terminator
  CorrectOut : Outport
  En_out : Outport  Port=2
  wires:
  AddSub3/1 -> Add1/1, CorrectOut/1
  Constant/1 -> AddSub3/1
  Temp/1 -> AddSub1/1
  Temp_c/1 -> AddSub1/2
  AddSub1/1 -> Add0/1, Mult3/2
  CoefTemp/1 -> Mult3/1
  Mult3/1 -> AddSub3/2, Mlt0/1
  en_in/1 -> Delay1/1, AddSub1/3
  Delay1/1 -> Delay2/1
  Delay2/1 -> Delay3/1, AddSub3/3
  Delay3/1 -> En_out/1
  Add0/1 -> Terminator/1
  Add1/1 -> Terminator1/1
  Mlt0/1 -> Terminator2/1

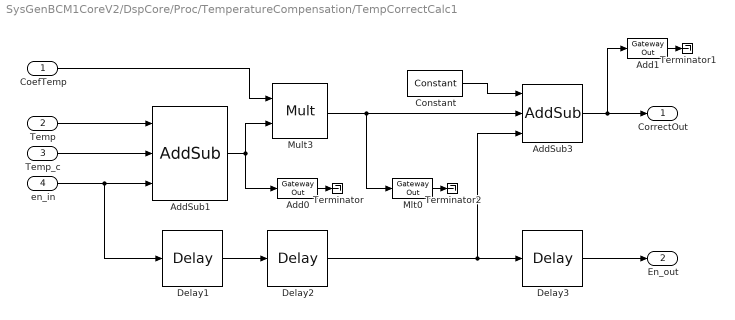
== system SysGenBCM1CoreV2/DspCore/Proc/TemperatureCompensation/TempCorrectCalc1 ==
  CoefTemp : Inport
  Temp : Inport  Port=2
  Temp_c : Inport  Port=3
  en_in : Inport  Port=4
  Add0 : xbsIndex_r4/Gateway Out  inherit_from_input=on  hdl_port=on  rows=1  columns=1  UseAsDAC=off  DACChannel='1'  interface=AXI4-Lite  automatic_assignment=off  address_offset=hex2dec('128')  intf_name=''  intf_description=''  timing_constraint=None  locs_specified=off  LOCs={}  io_standard={}  block_type=gatewayout
  Add1 : xbsIndex_r4/Gateway Out  inherit_from_input=on  hdl_port=on  rows=1  columns=1  UseAsDAC=off  DACChannel='1'  interface=AXI4-Lite  automatic_assignment=off  address_offset=hex2dec('130')  intf_name=''  intf_description=''  timing_constraint=None  locs_specified=off  LOCs={}  io_standard={}  block_type=gatewayout
  AddSub1 : xbsIndex_r4/AddSub  mode=Subtraction  use_carryin=off  use_carryout=off  en=on  latency=3  precision=Full  arith_type=Unsigned  n_bits=16  bin_pt=14  quantization=Truncate  overflow=Wrap  use_behavioral_HDL=off  hw_selection=Fabric  pipelined=off  dbl_ovrd=off  block_type=addsub
  AddSub3 : xbsIndex_r4/AddSub  mode=Addition  use_carryin=off  use_carryout=off  en=on  latency=2  precision=Full  arith_type=Unsigned  n_bits=16  bin_pt=14  quantization=Truncate  overflow=Wrap  use_behavioral_HDL=off  hw_selection=Fabric  pipelined=off  dbl_ovrd=off  block_type=addsub
  Constant : xbsIndex_r4/Constant  const=1.0  gui_display_data_type=Floating-point  arith_type=Floating-point  n_bits=16  bin_pt=14  preci_type=Single  exp_width=8  frac_width=24  explicit_period=off  period=1  equ=P=C  opselect=C  inp2=PCIN>>17  opr=+  inp1=P  carry=CIN  dbl_ovrd=off  block_type=constant
  Delay1 : xbsIndex_r4/Delay  rst=off  infoeditControl=Selection of Reset will increase slice count due to use of real FFs and instead of SRLs  en=off  latency=3  reg_retiming=off  dbl_ovrd=off  block_type=delay
      settings: infoedit=Hardware notes: A delay line is a chain, each link of which is an SRL16 or SRL32 followed by a flip-flop.
  Delay2 : xbsIndex_r4/Delay  rst=off  infoeditControl=Selection of Reset will increase slice count due to use of real FFs and instead of SRLs  en=off  latency=4  reg_retiming=off  dbl_ovrd=off  block_type=delay
      settings: infoedit=Hardware notes: A delay line is a chain, each link of which is an SRL16 or SRL32 followed by a flip-flop.
  Delay3 : xbsIndex_r4/Delay  rst=off  infoeditControl=Selection of Reset will increase slice count due to use of real FFs and instead of SRLs  en=off  latency=2  reg_retiming=off  dbl_ovrd=off  block_type=delay
      settings: infoedit=Hardware notes: A delay line is a chain, each link of which is an SRL16 or SRL32 followed by a flip-flop.
  Mlt0 : xbsIndex_r4/Gateway Out  inherit_from_input=on  hdl_port=on  rows=1  columns=1  UseAsDAC=off  DACChannel='1'  interface=AXI4-Lite  automatic_assignment=off  address_offset=hex2dec('12c')  intf_name=''  intf_description=''  timing_constraint=None  locs_specified=off  LOCs={}  io_standard={}  block_type=gatewayout
  Mult3 : xbsIndex_r4/Mult  precision=Full  arith_type="Signed  (2's comp)"  n_bits=16  bin_pt=14  quantization=Truncate  overflow=Wrap  en=off  latency=4  use_behavioral_HDL=off  opt=Speed  use_embedded=on  optimum_pipeline=off  pipeline=on  dbl_ovrd=off  use_rpm=on  placement_style=Triangular  block_type=mult
  Terminator : Terminator
  Terminator1 : Terminator
  Terminator2 : Terminator
  CorrectOut : Outport
  En_out : Outport  Port=2
  wires:
  AddSub3/1 -> Add1/1, CorrectOut/1
  Constant/1 -> AddSub3/1
  Temp/1 -> AddSub1/1
  Temp_c/1 -> AddSub1/2
  AddSub1/1 -> Add0/1, Mult3/2
  CoefTemp/1 -> Mult3/1
  Mult3/1 -> AddSub3/2, Mlt0/1
  en_in/1 -> Delay1/1, AddSub1/3
  Delay1/1 -> Delay2/1
  Delay2/1 -> Delay3/1, AddSub3/3
  Delay3/1 -> En_out/1
  Add0/1 -> Terminator/1
  Add1/1 -> Terminator1/1
  Mlt0/1 -> Terminator2/1

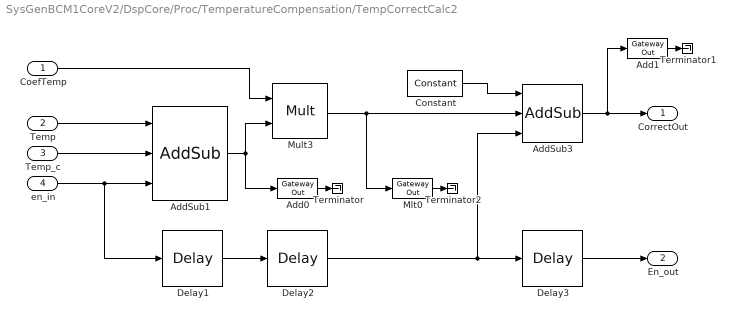
== system SysGenBCM1CoreV2/DspCore/Proc/TemperatureCompensation/TempCorrectCalc2 ==
  CoefTemp : Inport
  Temp : Inport  Port=2
  Temp_c : Inport  Port=3
  en_in : Inport  Port=4
  Add0 : xbsIndex_r4/Gateway Out  inherit_from_input=on  hdl_port=on  rows=1  columns=1  UseAsDAC=off  DACChannel='1'  interface=AXI4-Lite  automatic_assignment=off  address_offset=hex2dec('134')  intf_name=''  intf_description=''  timing_constraint=None  locs_specified=off  LOCs={}  io_standard={}  block_type=gatewayout
  Add1 : xbsIndex_r4/Gateway Out  inherit_from_input=on  hdl_port=on  rows=1  columns=1  UseAsDAC=off  DACChannel='1'  interface=AXI4-Lite  automatic_assignment=off  address_offset=hex2dec('13C')  intf_name=''  intf_description=''  timing_constraint=None  locs_specified=off  LOCs={}  io_standard={}  block_type=gatewayout
  AddSub1 : xbsIndex_r4/AddSub  mode=Subtraction  use_carryin=off  use_carryout=off  en=on  latency=3  precision=Full  arith_type=Unsigned  n_bits=16  bin_pt=14  quantization=Truncate  overflow=Wrap  use_behavioral_HDL=off  hw_selection=Fabric  pipelined=off  dbl_ovrd=off  block_type=addsub
  AddSub3 : xbsIndex_r4/AddSub  mode=Addition  use_carryin=off  use_carryout=off  en=on  latency=2  precision=Full  arith_type=Unsigned  n_bits=16  bin_pt=14  quantization=Truncate  overflow=Wrap  use_behavioral_HDL=off  hw_selection=Fabric  pipelined=off  dbl_ovrd=off  block_type=addsub
  Constant : xbsIndex_r4/Constant  const=1.0  gui_display_data_type=Floating-point  arith_type=Floating-point  n_bits=16  bin_pt=14  preci_type=Single  exp_width=8  frac_width=24  explicit_period=off  period=1  equ=P=C  opselect=C  inp2=PCIN>>17  opr=+  inp1=P  carry=CIN  dbl_ovrd=off  block_type=constant
  Delay1 : xbsIndex_r4/Delay  rst=off  infoeditControl=Selection of Reset will increase slice count due to use of real FFs and instead of SRLs  en=off  latency=3  reg_retiming=off  dbl_ovrd=off  block_type=delay
      settings: infoedit=Hardware notes: A delay line is a chain, each link of which is an SRL16 or SRL32 followed by a flip-flop.
  Delay2 : xbsIndex_r4/Delay  rst=off  infoeditControl=Selection of Reset will increase slice count due to use of real FFs and instead of SRLs  en=off  latency=4  reg_retiming=off  dbl_ovrd=off  block_type=delay
      settings: infoedit=Hardware notes: A delay line is a chain, each link of which is an SRL16 or SRL32 followed by a flip-flop.
  Delay3 : xbsIndex_r4/Delay  rst=off  infoeditControl=Selection of Reset will increase slice count due to use of real FFs and instead of SRLs  en=off  latency=2  reg_retiming=off  dbl_ovrd=off  block_type=delay
      settings: infoedit=Hardware notes: A delay line is a chain, each link of which is an SRL16 or SRL32 followed by a flip-flop.
  Mlt0 : xbsIndex_r4/Gateway Out  inherit_from_input=on  hdl_port=on  rows=1  columns=1  UseAsDAC=off  DACChannel='1'  interface=AXI4-Lite  automatic_assignment=off  address_offset=hex2dec('138')  intf_name=''  intf_description=''  timing_constraint=None  locs_specified=off  LOCs={}  io_standard={}  block_type=gatewayout
  Mult3 : xbsIndex_r4/Mult  precision=Full  arith_type="Signed  (2's comp)"  n_bits=16  bin_pt=14  quantization=Truncate  overflow=Wrap  en=off  latency=4  use_behavioral_HDL=off  opt=Speed  use_embedded=on  optimum_pipeline=off  pipeline=on  dbl_ovrd=off  use_rpm=on  placement_style=Triangular  block_type=mult
  Terminator : Terminator
  Terminator1 : Terminator
  Terminator2 : Terminator
  CorrectOut : Outport
  En_out : Outport  Port=2
  wires:
  AddSub3/1 -> Add1/1, CorrectOut/1
  Constant/1 -> AddSub3/1
  Temp/1 -> AddSub1/1
  Temp_c/1 -> AddSub1/2
  AddSub1/1 -> Add0/1, Mult3/2
  CoefTemp/1 -> Mult3/1
  Mult3/1 -> AddSub3/2, Mlt0/1
  en_in/1 -> Delay1/1, AddSub1/3
  Delay1/1 -> Delay2/1
  Delay2/1 -> Delay3/1, AddSub3/3
  Delay3/1 -> En_out/1
  Add0/1 -> Terminator/1
  Add1/1 -> Terminator1/1
  Mlt0/1 -> Terminator2/1
